simulink model "EZQStEnCtrl_logic"  (R2018b)
settings: Solver=VariableStepAuto  StartTime=0.0  StopTime=10.0  RelTol=1e-3
settings Model: Creator=sn2xws  LastModifiedBy=sn2xws

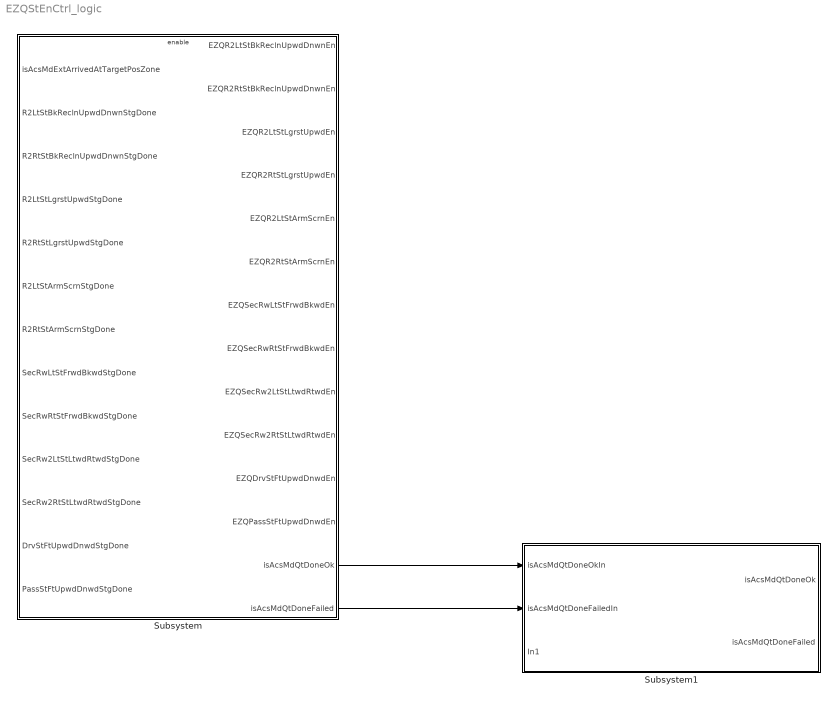
== system EZQStEnCtrl_logic ==
  Subsystem : Subsystem
  Subsystem1 : Subsystem
  wires:
  Subsystem/13(isAcsMdQtDoneOk) -> Subsystem1/1(isAcsMdQtDoneOkIn)
  Subsystem/14(isAcsMdQtDoneFailed) -> Subsystem1/2(isAcsMdQtDoneFailedIn)

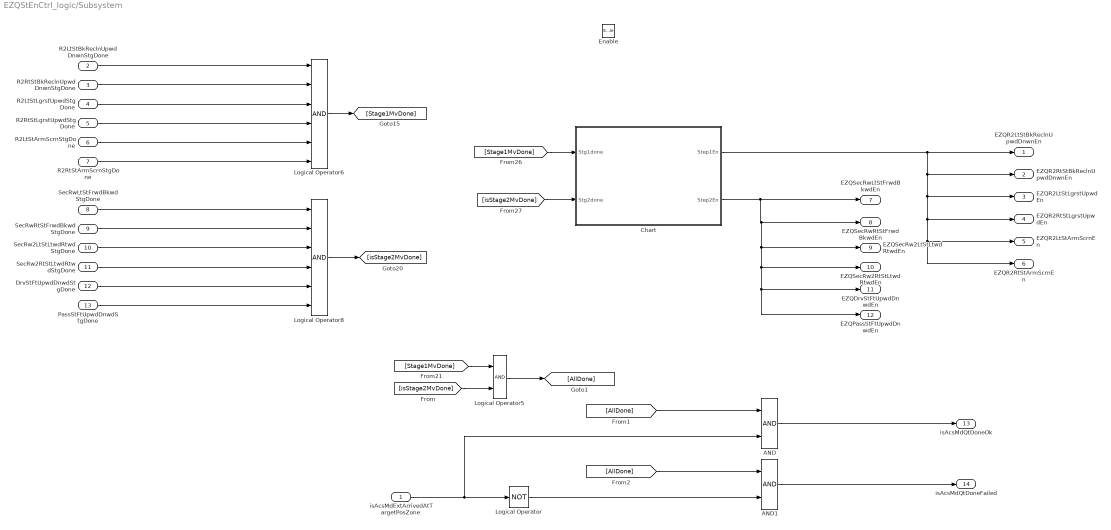
== system EZQStEnCtrl_logic/Subsystem ==
  isAcsMdExtArrivedAtTargetPosZone : Inport
  R2LtStBkReclnUpwdDnwnStgDone : Inport  Port=2
  R2RtStBkReclnUpwdDnwnStgDone : Inport  Port=3
  R2LtStLgrstUpwdStgDone : Inport  Port=4
  R2RtStLgrstUpwdStgDone : Inport  Port=5
  R2LtStArmScrnStgDone : Inport  Port=6
  R2RtStArmScrnStgDone : Inport  Port=7
  SecRwLtStFrwdBkwdStgDone : Inport  Port=8
  SecRwRtStFrwdBkwdStgDone : Inport  Port=9
  SecRw2LtStLtwdRtwdStgDone : Inport  Port=10
  SecRw2RtStLtwdRtwdStgDone : Inport  Port=11
  DrvStFtUpwdDnwdStgDone : Inport  Port=12
  PassStFtUpwdDnwdStgDone : Inport  Port=13
  Enable : EnablePort  StatesWhenEnabling=reset
  AND : Logic  AllPortsSameDT=off  OutDataTypeStr=boolean
  AND1 : Logic  AllPortsSameDT=off  OutDataTypeStr=boolean
  Chart : Stateflow chart  TreatAsAtomicUnit=on
  Logical Operator : Logic  Operator=NOT  AllPortsSameDT=off  OutDataTypeStr=boolean
  Logical Operator5 : Logic  AllPortsSameDT=off  OutDataTypeStr=boolean
  Logical Operator6 : Logic  Inputs=6  AllPortsSameDT=off  OutDataTypeStr=boolean
  Logical Operator8 : Logic  Inputs=6  AllPortsSameDT=off  OutDataTypeStr=boolean
  EZQR2LtStBkReclnUpwdDnwnEn : Outport
  EZQR2RtStBkReclnUpwdDnwnEn : Outport  Port=2
  EZQR2LtStLgrstUpwdEn : Outport  Port=3
  EZQR2RtStLgrstUpwdEn : Outport  Port=4
  EZQR2LtStArmScrnEn : Outport  Port=5
  EZQR2RtStArmScrnEn : Outport  Port=6
  EZQSecRwLtStFrwdBkwdEn : Outport  Port=7
  EZQSecRwRtStFrwdBkwdEn : Outport  Port=8
  EZQSecRw2LtStLtwdRtwdEn : Outport  Port=9
  EZQSecRw2RtStLtwdRtwdEn : Outport  Port=10
  EZQDrvStFtUpwdDnwdEn : Outport  Port=11
  EZQPassStFtUpwdDnwdEn : Outport  Port=12
  isAcsMdQtDoneOk : Outport  Port=13
  isAcsMdQtDoneFailed : Outport  Port=14
  wires:
  Logical Operator/1 -> AND1/2
  [AllDone] -> AND1/1
  Chart/2(Step2En) -> EZQSecRwLtStFrwdBkwdEn/1, EZQSecRwRtStFrwdBkwdEn/1, EZQSecRw2LtStLtwdRtwdEn/1, EZQSecRw2RtStLtwdRtwdEn/1, EZQPassStFtUpwdDnwdEn/1, EZQDrvStFtUpwdDnwdEn/1
  [isStage2MvDone] -> Logical Operator5/2
  Chart/1(Step1En) -> EZQR2LtStBkReclnUpwdDnwnEn/1, EZQR2RtStBkReclnUpwdDnwnEn/1, EZQR2LtStLgrstUpwdEn/1, EZQR2RtStLgrstUpwdEn/1, EZQR2RtStArmScrnEn/1, EZQR2LtStArmScrnEn/1
  SecRwRtStFrwdBkwdStgDone/1 -> Logical Operator8/2
  R2LtStBkReclnUpwdDnwnStgDone/1 -> Logical Operator6/1
  R2RtStBkReclnUpwdDnwnStgDone/1 -> Logical Operator6/2
  [isStage2MvDone] -> Chart/2(Stg2done)
  Logical Operator6/1 -> [Stage1MvDone]
  [AllDone] -> AND/1
  isAcsMdExtArrivedAtTargetPosZone/1 -> AND/2, Logical Operator/1
  R2LtStArmScrnStgDone/1 -> Logical Operator6/5
  [Stage1MvDone] -> Logical Operator5/1
  [Stage1MvDone] -> Chart/1(Stg1done)
  AND/1 -> isAcsMdQtDoneOk/1
  R2RtStLgrstUpwdStgDone/1 -> Logical Operator6/4
  Logical Operator5/1 -> [AllDone]
  SecRw2LtStLtwdRtwdStgDone/1 -> Logical Operator8/3
  R2LtStLgrstUpwdStgDone/1 -> Logical Operator6/3
  Logical Operator8/1 -> [isStage2MvDone]
  SecRwLtStFrwdBkwdStgDone/1 -> Logical Operator8/1
  R2RtStArmScrnStgDone/1 -> Logical Operator6/6
  SecRw2RtStLtwdRtwdStgDone/1 -> Logical Operator8/4
  AND1/1 -> isAcsMdQtDoneFailed/1
  PassStFtUpwdDnwdStgDone/1 -> Logical Operator8/6
  DrvStFtUpwdDnwdStgDone/1 -> Logical Operator8/5

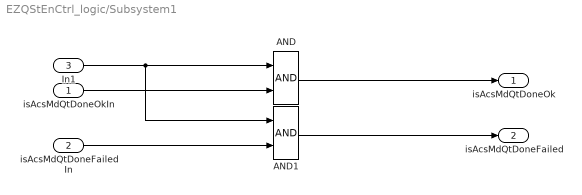
== system EZQStEnCtrl_logic/Subsystem1 ==
  isAcsMdQtDoneOkIn : Inport
  isAcsMdQtDoneFailedIn : Inport  Port=2
  In1 : Inport  Port=3
  AND : Logic  AllPortsSameDT=off  OutDataTypeStr=boolean
  AND1 : Logic  AllPortsSameDT=off  OutDataTypeStr=boolean
  isAcsMdQtDoneOk : Outport
  isAcsMdQtDoneFailed : Outport  Port=2
  wires:
  isAcsMdQtDoneOkIn/1 -> AND/2
  AND1/1 -> isAcsMdQtDoneFailed/1
  In1/1 -> AND1/1, AND/1
  AND/1 -> isAcsMdQtDoneOk/1
  isAcsMdQtDoneFailedIn/1 -> AND1/2

== stateflow chart EZQStEnCtrl_logic/Subsystem/Chart ==
  (default) -> (junction 58)
  (junction 58) -> (junction 25) [order 1] : [Stg1done]
  (junction 58) -> (junction 35) [order 2] : {Stg1Req=true;}
  (junction 25) -> (junction 18) : {
      | Stg1Req=false;
      | }
  (junction 18) -> (junction 35)
  (junction 35) -> (junction 44)
  (junction 44) -> (junction 33) [order 1] : [Stg2done]
  (junction 44) -> (junction 45) [order 2] : {
      | Stg2Req=true;
      | }
  (junction 33) -> (junction 73) : {
      | Stg2Req=false;
      | }
  (junction 73) -> (junction 45)
  (junction 45) -> (junction 31)
  (junction 31) -> (junction 34) [order 1] : [Stg1Req==true]
  (junction 31) -> (junction 38) [order 2]
  (junction 34) -> (junction 47) : {
      | Step1En = true;
      | Step2En = false;
      | }
  (junction 38) -> (junction 24) [order 1] : [Stg2Req==true]
  (junction 38) -> (junction 71) [order 2] : {
      | Step1En = false;
      | Step2En = false;
      | }
  (junction 24) -> (junction 72) : {
      | Step1En = false;
      | Step2En = true;
      | }
  (junction 72) -> (junction 71)
  (junction 47) -> (junction 72)
  (junction 71) -> (junction 48)
  data: Stg1done input boolean; Stg2done input boolean; Step1En output boolean; Step2En output boolean; Stg1Req local boolean; Stg2Req local boolean
